simulink model "VFD"  (R2016a)
settings: Solver=FixedStepDiscrete  StartTime=0.0  StopTime=4  FixedStep=5e-6  RelTol=1e-3
undefined symbols (not defined in the file): DiscIntNeverNeededParam, infinite
libraries: powerlib x12, powerlib_meascontrol x2
settings Model: Creator=ASUS  LastModifiedBy=ASUS
settings DebuggingCC: UnconnectedInputMsg=none  UnconnectedOutputMsg=none  UnconnectedLineMsg=none

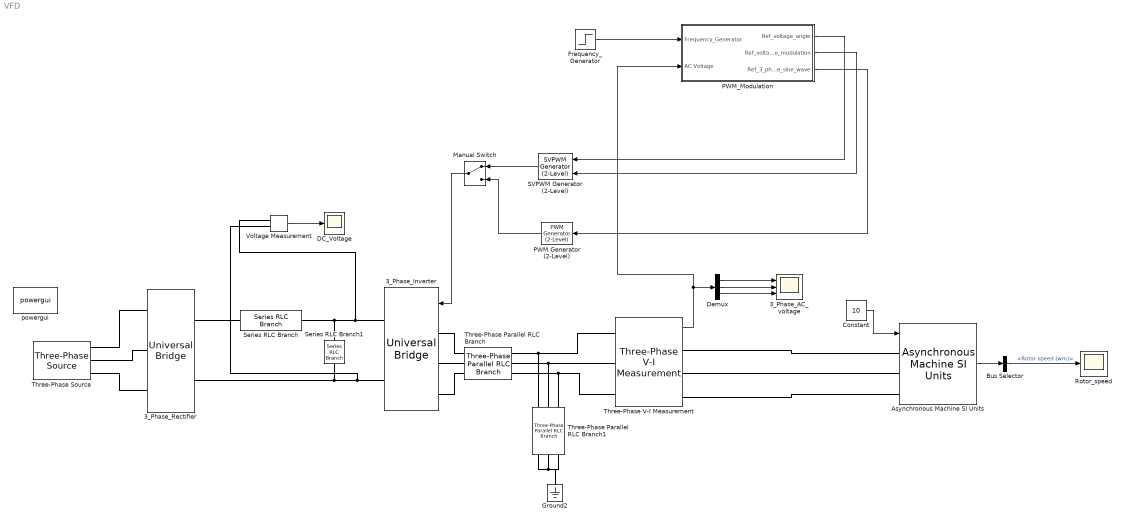
== system VFD ==
  3_Phase_AC_voltage : Scope  NumInputPorts=3
  3_Phase_Inverter : powerlib/Power Electronics/Universal Bridge  Arms=3  SnubberResistance=1e5  SnubberCapacitance=inf  Device=IGBT / Diodes  Ron=1e-3  Lon=0  ForwardVoltages="[  0  0  ]"  ForwardVoltage=0  GTOparameters=[ 10e-6 , 20e-6 ]  IGBTparameters=[ 1e-6 , 2e-6 ]  Measurements=UAB UBC UCA UDC voltages  Measurements_2=None  converterType=Rectifier
  3_Phase_Rectifier : powerlib/Power Electronics/Universal Bridge  Arms=3  SnubberResistance=1e5  SnubberCapacitance=inf  Device=Diodes  Ron=1e-3  Lon=0  ForwardVoltages="[  0  0  ]"  ForwardVoltage=0  GTOparameters=[ 10e-6 , 20e-6 ]  IGBTparameters=[ 1e-6 , 2e-6 ]  Measurements=None  Measurements_2=None  converterType=Rectifier
  Asynchronous Machine SI Units : powerlib/Machines/Asynchronous Machine SI Units  RotorType=Squirrel-cage  PresetModel=No  MechanicalLoad=Torque Tm  ShowDetailedParameters=on  ReferenceFrame=Rotor  Units=SI  MeasurementBus=off  NominalParameters=[1.845e+04 400 50]  Stator=[0.5968 0.0003495]  Rotor=[0.6258 0.005473]  Cage1=[0.4155 0.002066]  Cage2=[0.4168 0.0003495]  Lm=0.0354  Mechanical=[0.05 0.005879 2]  PolePairs=2  InitialConditions=[0 0 0 0 0 0 0 0]  SimulateSaturation=off  Saturation=[14.03593122, 27.81365428, 53.79336849, 72.68890987, 97.98006896, 148.6815601, 215.7428561, 302.9841135, 428.7778367 ; 230, 322, 414, 460, 506, 552, 598, 644, 690]  LoadFlowParameters=1492000  TsPowergui=0  TsBlock=-1  IterativeModel=Trapezoidal non iterative  IterativeDiscreteModel=Trapezoidal non iterative  Pmec=1.492e+006
  Bus Selector : BusSelector  OutputSignals=Mechanical.Rotor speed (wm)
  Constant : Constant  Value=10
  DC_Voltage : Scope
  Demux : Demux  Outputs=3
  Frequency_Generator : Step  Before=50  After=10  SampleTime=0
  Ground2 : powerlib/Elements/Ground  LConnTagsString=a
  Manual Switch : ManualSwitch
  PWM Generator (2-Level) : powerlib_meascontrol/Pulse & Signal Generators/PWM Generator (2-Level)  ModulatorType=Three-phase bridge (6 pulses)  ModulatorMode=Unsynchronized  Fc=10000  Pc=90  nF=27  MinMax="[ -1  1 ]"  SamplingTechnique=Natural  ModulatingSignals=off  m=0.8  Freq=50  Phase=0  Ts=0  ShowCarrierOutport=off
  "PWM_Modulation " : Subsystem
  Rotor_speed : Scope
  SVPWM Generator (2-Level) : powerlib_meascontrol/Pulse & Signal Generators/SVPWM Generator (2-Level)  InputType=Magnitude-Angle (rad)  SwitchingPattern=Pattern #1  Fc=5000  ParUref=[0.8 -30 50]  Ts=5e-6
  Series RLC Branch : powerlib/Elements/Series RLC Branch  LConnTagsString=__new0  RConnTagsString=__new0  BranchType=L  Resistance=1  Inductance=5e-3  SetiL0=off  InitialCurrent=0  Capacitance=infinite  Setx0=off  InitialVoltage=0  Measurements=None
  Series RLC Branch1 : powerlib/Elements/Series RLC Branch  LConnTagsString=__new0  RConnTagsString=__new0  BranchType=C  Resistance=1  Inductance=5e-3  SetiL0=off  InitialCurrent=0  Capacitance=2200e-6  Setx0=off  InitialVoltage=0  Measurements=None
  Three-Phase Parallel RLC Branch : powerlib/Elements/Three-Phase Parallel RLC Branch  LConnTagsString=A|B|C  RConnTagsString=A|B|C  BranchType=RL  Resistance=0.2  Inductance=0.1e-3  Capacitance=1e-6  Measurements=None
  Three-Phase Parallel RLC Branch1 : powerlib/Elements/Three-Phase Parallel RLC Branch  LConnTagsString=A|B|C  RConnTagsString=A|B|C  BranchType=C  Resistance=1  Inductance=1e-3  Capacitance=600e-6  Measurements=None
  Three-Phase V-I Measurement : powerlib/Measurements/Three-Phase V-I Measurement  VoltageMeasurement=phase-to-phase  SetLabelV=off  LabelV=Vabc  Vpu=off  VpuLL=off  CurrentMeasurement=no  SetLabelI=off  LabelI=Iabc  Ipu=off  Pbase=100e6  Vbase=500e3  OutputType=Complex  PhasorSimulation=off  PSBequivalent=0
  Three-Phase Source : powerlib/Electrical Sources/Three-Phase Source  InternalConnection=Yg  VoltagePhases=off  Voltage=415  PhaseAngle=0  Voltage_phases=[25e3 25e3 25e3]/sqrt(3)  PhaseAngles_phases=[0 -120 +120]  Frequency=50  NonIdealSource=on  SpecifyImpedance=off  Resistance=0.01  Inductance=1e-3  ShortCircuitLevel=100e6  BaseVoltage=415  XRratio=7  BusType=swing  Pref=10e3  Qref=0  Prefabc=[10e3, 10e3, 10e3]  Qrefabc=[0, 0, 0]  Qmin=-inf  Qmax=inf
  Voltage Measurement : powerlib/Measurements/Voltage Measurement  PhasorSimulation=off  OutputType=Complex  PSBequivalent=0
  powergui : powerlib/powergui  Priority=1  SimulationMode=Discrete  SolverType=Tustin/Backward Euler (TBE)  SampleTime=5e-6  frequency=60  SPID=off  DisableSnubberDevices=off  DisableRonSwitches=off  DisableVfSwitches=off  SwTol=0  DisplayEquations=off  Interpol=off  ExternalGateDelay=off  methode=off  Ts=10  FunctionMessages=off  echomessages=off  HookPort=off  EnableUseOfTLC=off  x0status=blocks  frequencyindice=50  Pbase=100e6  ErrMax=1e-4  Iterations=50  UnitsV=kV  UnitsW=MW  buscounter=0  RestoreLinks=warning  ResistiveCurrentMeasurement=off  Frange=[0:2:500]  Ylog=off  Xlog=on  ShowGrid=off  save=off  variable=ZData  structure=0  ZoomFFT=off  StartTime=0.0  cycles=1  DisplayStyle=1  fundamental=60  FreqAxis=off  MaxFrequency=1000  frequencyindicesteady=1  RmsSteady=1  display=off
  wires:
  Constant/1 -> Asynchronous Machine SI Units/1
  Asynchronous Machine SI Units/1 -> Bus Selector/1
  Bus Selector/1 -> Rotor_speed/1  "<Rotor speed (wm)>"
  Voltage Measurement/1 -> DC_Voltage/1
  Demux/1 -> 3_Phase_AC_voltage/1
  Demux/2 -> 3_Phase_AC_voltage/2
  Demux/3 -> 3_Phase_AC_voltage/3
  Three-Phase V-I Measurement/1 -> "PWM_Modulation "/2(AC Voltage), Demux/1
  SVPWM Generator (2-Level)/1 -> Manual Switch/1
  PWM Generator (2-Level)/1 -> Manual Switch/2
  Manual Switch/1 -> 3_Phase_Inverter/1
  Frequency_Generator/1 -> "PWM_Modulation "/1(Frequency_Generator)
  "PWM_Modulation "/1(Ref_voltage_angle) -> SVPWM Generator (2-Level)/2
  "PWM_Modulation "/2(Ref_voltage_modulation) -> SVPWM Generator (2-Level)/1
  "PWM_Modulation "/3(Ref_3_phase_sine_wave) -> PWM Generator (2-Level)/1
  connections:
  Three-Phase Source/RConn1 -- 3_Phase_Rectifier/LConn1
  Three-Phase Source/RConn3 -- 3_Phase_Rectifier/LConn3
  Three-Phase Source/RConn2 -- 3_Phase_Rectifier/LConn2
  3_Phase_Rectifier/RConn1 -- Series RLC Branch/LConn1
  Series RLC Branch/RConn1 -- Series RLC Branch1/LConn1 -- Voltage Measurement/LConn1 -- 3_Phase_Inverter/RConn1
  3_Phase_Rectifier/RConn2 -- Series RLC Branch1/RConn1 -- Voltage Measurement/LConn2 -- 3_Phase_Inverter/RConn2
  Three-Phase Parallel RLC Branch/LConn2 -- 3_Phase_Inverter/LConn2
  3_Phase_Inverter/LConn1 -- Three-Phase Parallel RLC Branch/LConn1
  3_Phase_Inverter/LConn3 -- Three-Phase Parallel RLC Branch/LConn3
  Three-Phase Parallel RLC Branch/RConn1 -- Three-Phase Parallel RLC Branch1/LConn1 -- Three-Phase V-I Measurement/LConn1
  Three-Phase Parallel RLC Branch/RConn2 -- Three-Phase Parallel RLC Branch1/LConn2 -- Three-Phase V-I Measurement/LConn2
  Three-Phase Parallel RLC Branch/RConn3 -- Three-Phase Parallel RLC Branch1/LConn3 -- Three-Phase V-I Measurement/LConn3
  Three-Phase Parallel RLC Branch1/RConn2 -- Three-Phase Parallel RLC Branch1/RConn3 -- Ground2/LConn1 -- Three-Phase Parallel RLC Branch1/RConn1
  Asynchronous Machine SI Units/LConn1 -- Three-Phase V-I Measurement/RConn1
  Three-Phase V-I Measurement/RConn2 -- Asynchronous Machine SI Units/LConn2
  Asynchronous Machine SI Units/LConn3 -- Three-Phase V-I Measurement/RConn3

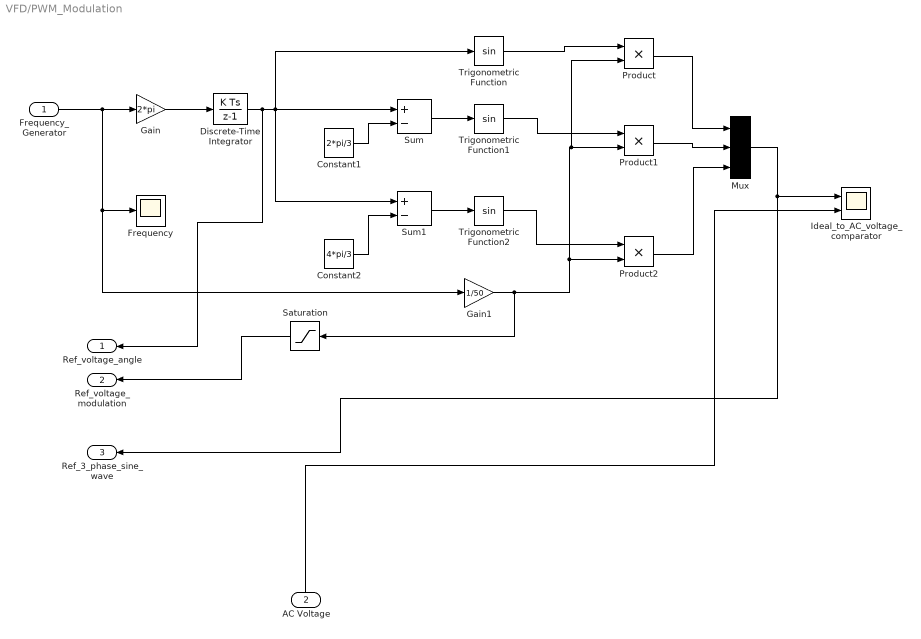
== system VFD/PWM_Modulation  ==
  Frequency_Generator : Inport
  AC Voltage : Inport  Port=2
  Constant1 : Constant  Value=2*pi/3
  Constant2 : Constant  Value=4*pi/3
  Discrete-Time Integrator : DiscreteIntegrator  InitialConditionSetting=State (most efficient)  SampleTime=5e-6  ICPrevOutput=DiscIntNeverNeededParam  ICPrevScaledInput=DiscIntNeverNeededParam
  Frequency : Scope
  Gain : Gain  Gain=2*pi
  Gain1 : Gain  Gain=1/50
  Ideal_to_AC_voltage_comparator : Scope  NumInputPorts=2
  Mux : Mux  Inputs=3
  Product : Product
  Product1 : Product
  Product2 : Product
  Saturation : Saturate  UpperLimit=1  LowerLimit=0
  Sum : Sum  Inputs=+-
  Sum1 : Sum  Inputs=+-
  Trigonometric Function : Trigonometry
  Trigonometric Function1 : Trigonometry
  Trigonometric Function2 : Trigonometry
  Ref_voltage_angle : Outport
  Ref_voltage_modulation : Outport  Port=2
  Ref_3_phase_sine_wave : Outport  Port=3
  wires:
  AC Voltage/1 -> Ideal_to_AC_voltage_comparator/2
  Trigonometric Function1/1 -> Product1/1
  Constant1/1 -> Sum/2
  Constant2/1 -> Sum1/2
  Discrete-Time Integrator/1 -> Ref_voltage_angle/1, Sum1/1, Trigonometric Function/1, Sum/1
  Product2/1 -> Mux/3
  Mux/1 -> Ref_3_phase_sine_wave/1, Ideal_to_AC_voltage_comparator/1
  Product1/1 -> Mux/2
  Trigonometric Function2/1 -> Product2/1
  Gain1/1 -> Saturation/1, Product/2, Product1/2, Product2/2
  Trigonometric Function/1 -> Product/1
  Gain/1 -> Discrete-Time Integrator/1
  Frequency_Generator/1 -> Frequency/1, Gain1/1, Gain/1
  Product/1 -> Mux/1
  Saturation/1 -> Ref_voltage_modulation/1
  Sum/1 -> Trigonometric Function1/1
  Sum1/1 -> Trigonometric Function2/1
